simulink model "kolo_popov"  (R2022b)
settings: Solver=VariableStepAuto  StartTime=0.0  StopTime=T  RelTol=1e-3
undefined symbols (not defined in the file): A, b, c, M
settings Model: Creator=Andrzej  LastModifiedBy=Andrzej

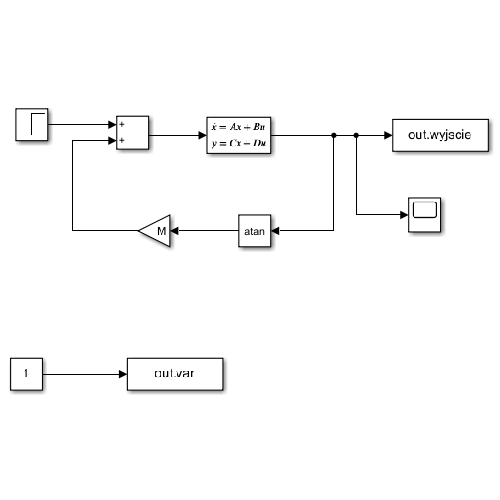
[thumbnail: Simulink's stored preview of the top-level diagram]
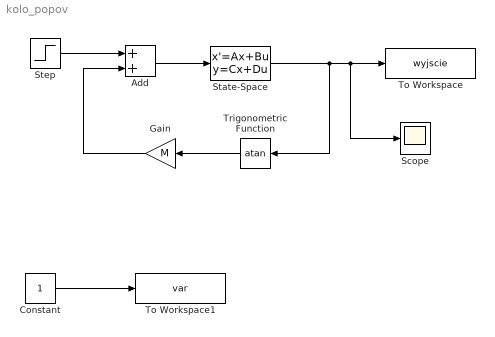
== system kolo_popov ==
  Add : Sum
  Constant : Constant
  Gain : Gain  Gain=M
  Scope : Scope
  State-Space : StateSpace  A=A  B=b  C=c  D=[0]  InitialCondition=0
  Step : Step  Time=0  SampleTime=0
  To Workspace : ToWorkspace  VariableName=wyjscie  SampleTime=-1
      settings: Save2DSignal=2-D array (concatenate along first dimension)
  To Workspace1 : ToWorkspace  VariableName=var  SaveFormat=Timeseries  SampleTime=-1
  Trigonometric Function : Trigonometry  Operator=atan
  wires:
  Gain/1 -> Add/2
  State-Space/1 -> Scope/1, To Workspace/1, Trigonometric Function/1
  Add/1 -> State-Space/1
  Trigonometric Function/1 -> Gain/1
  Step/1 -> Add/1
  Constant/1 -> To Workspace1/1
